simulink model "sparse_learning_recalling"  (R2021b)
settings: Solver=FixedStepDiscrete  StartTime=0.0  StopTime=200.0  FixedStep=0.5  RelTol=1e-3
libraries: wnnlib x7
settings Model: Creator=20214358  LastModifiedBy=20214358

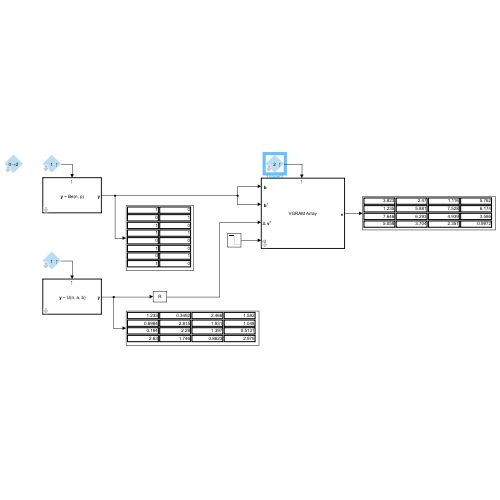
[thumbnail: Simulink's stored preview of the top-level diagram]
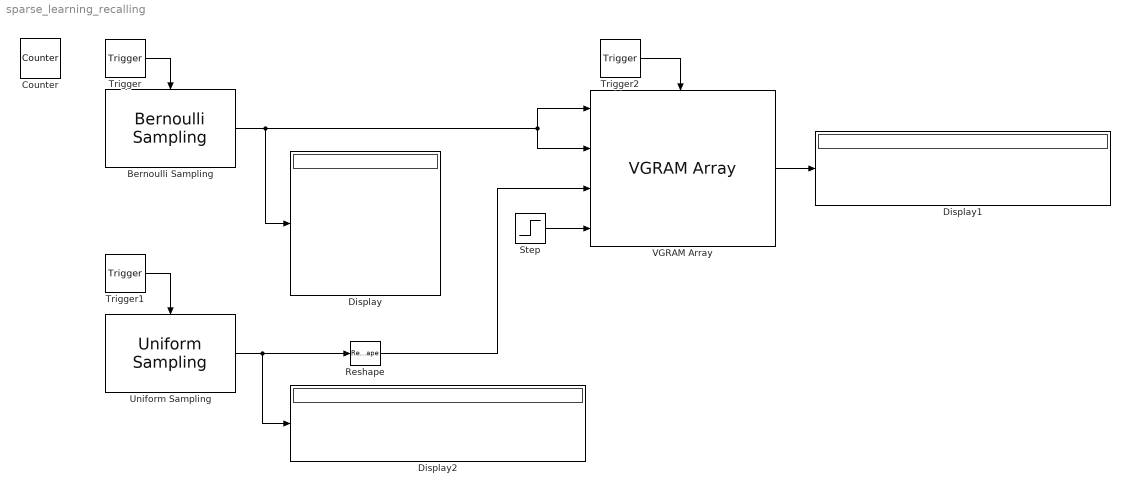
== system sparse_learning_recalling ==
  Bernoulli Sampling : wnnlib/Sources/Bernoulli Sampling  nSamples=16  probability=0.5  nSeed=0
      settings: SourceProductName=Weightless Neural Networks Toolbox
  Counter : wnnlib/Sources/Counter  number_of_steps=2  sample_time=-1
      settings: SourceProductName=Weightless Neural Networks Toolbox
  Display : Display
  Display1 : Display
  Display2 : Display
  Reshape : Reshape  OutputDimensionality=Customize  OutputDimensions=[4,4]
  Step : Step  Time=100  Before=1  After=0  OutDataTypeStr=Inherit: Inherit via back propagation  SampleTime=0.5
  Trigger : wnnlib/Sources/Trigger  selected_steps=1
      settings: SourceProductName=Weightless Neural Networks Toolbox
  Trigger1 : wnnlib/Sources/Trigger  selected_steps=1
      settings: SourceProductName=Weightless Neural Networks Toolbox
  Trigger2 : wnnlib/Sources/Trigger  selected_steps=2
      settings: SourceProductName=Weightless Neural Networks Toolbox
  Uniform Sampling : wnnlib/Sources/Uniform Sampling  nSamples=16  min_value=0  max_value=3  nSeed=1
      settings: SourceProductName=Weightless Neural Networks Toolbox
  VGRAM Array : wnnlib/Models/VGRAM Array  array_id=0  min_mem_size=65535  max_mem_size=65536  min_dist=2  max_dist=8  pattern_length=16  output_dims=[4, 4]  debug_flag=on
      settings: SourceProductName=Weightless Neural Networks Toolbox
  wires:
  Bernoulli Sampling/1 -> VGRAM Array/2, VGRAM Array/1, Display/1
  VGRAM Array/1 -> Display1/1
  Uniform Sampling/1 -> Reshape/1, Display2/1
  Step/1 -> VGRAM Array/4
  Reshape/1 -> VGRAM Array/3
  Trigger/1 -> Bernoulli Sampling/Trigger
  Trigger1/1 -> Uniform Sampling/Trigger
  Trigger2/1 -> VGRAM Array/Trigger
